simulink model "car_model"  (R2017a)
settings: Solver=VariableStepAuto  StartTime=0.0  StopTime=tf  RelTol=1e-3  AbsTol=1e-6
values from neighbouring files (symbols this model uses):
  MAX_DELTA_i = deg2rad(MAX_DELTA_i)    [run_sim.m]
  x0 = double(subs([qs0; ps0], symbs, vals))    [run_sim.m]
undefined symbols (not defined in the file or in its folder): sys
(part 2 of 2)

== matlab function car_model/Vehicle/Steering_model/Efforts/Constrained_efforts ==
  data: in1 input; in2 input; fs output
function fs = ConstrainedEffort(in1,in2)

%    This function was generated by the Symbolic Math Toolbox version 7.2.

%    28-Oct-2020 21:52:33



delta_i = in1(4,:);

delta_o = in1(5,:);

f_phi_i = in2(1,:);

f_phi_l = in2(4,:);

f_phi_o = in2(2,:);

f_phi_r = in2(3,:);

p1 = in1(10,:);

p2 = in1(11,:);

p3 = in1(12,:);

p4 = in1(13,:);

phi_i = in1(6,:);

phi_l = in1(9,:);

phi_o = in1(7,:);

phi_r = in1(8,:);

theta = in1(3,:);

t2 = p1.^2;

t3 = p4.^2;

t4 = theta.*2.0;

t5 = p3.^2;

t6 = delta_i.*2.0;

t7 = delta_o.*2.0;

t8 = phi_o.*2.0;

t9 = p2.^2;

t10 = t4+t7+t8;

t11 = sin(t10);

t12 = t4+t7-t8;

t13 = sin(t12);

t14 = phi_o.*4.0;

t15 = t4+t7+t14;

t16 = sin(t15);

t17 = sin(t4);

t18 = t4+t7;

t19 = sin(t18);

t20 = phi_l.*2.0;

t21 = phi_l.*4.0;

t22 = -t4+t20;

t23 = sin(t22);

t24 = t4+t20;

t25 = sin(t24);

t26 = phi_l.*3.0;

t27 = phi_r.*2.0;

t28 = phi_r.*4.0;

t29 = phi_i.*4.0;

t30 = delta_o-t14+theta;

t31 = sin(t30);

t32 = delta_o+t14+theta;

t33 = sin(t32);

t34 = phi_o.*3.0;

t35 = delta_o+theta;

t36 = sin(t35);

t37 = tan(delta_i);

t38 = t37.*(3.0./2.0);

t39 = t38+9.0./2.0;

t40 = 1.0./t39.^2;

t41 = t21+theta;

t42 = sin(t41);

t43 = t4+t7-t14;

t44 = sin(t43);

t45 = sin(t8);

t46 = sin(t14);

t47 = -t4+t27;

t48 = sin(t47);

t49 = t4+t27;

t50 = sin(t49);

t51 = phi_r.*3.0;

t52 = t21-theta;

t53 = sin(t52);

t54 = -t4+t21;

t55 = sin(t54);

t56 = t4+t21;

t57 = sin(t56);

t58 = cos(theta);

t59 = sin(theta);

t60 = phi_i.*2.0;

t64 = cos(t6);

t65 = t64.*(9.0./2.0);

t66 = sin(t6);

t67 = t66.*(3.0./2.0);

t61 = t65+t67+9.0./2.0;

t62 = t4+t6+t60;

t63 = sin(t62);

t68 = t61.^2;

t69 = cos(t7);

t70 = t69.*(9.0./2.0);

t71 = sin(t7);

t74 = t71.*(3.0./2.0);

t72 = t70-t74+9.0./2.0;

t73 = 1.0./t72.^2;

t75 = t4+t6+t29;

t76 = sin(t75);

t77 = t28+theta;

t78 = sin(t77);

t79 = t4+t6;

t80 = sin(t79);

t81 = delta_i-t29+theta;

t82 = sin(t81);

t83 = delta_i+t29+theta;

t84 = sin(t83);

t85 = 1.0./t39;

t86 = delta_i+theta;

t87 = sin(t86);

t88 = t28-theta;

t89 = sin(t88);

t90 = -t4+t28;

t91 = sin(t90);

t92 = t4+t28;

t93 = sin(t92);

t94 = 1.0./t72;

t95 = t4+t6-t60;

t96 = sin(t95);

t97 = t4+t6-t29;

t98 = sin(t97);

t99 = cos(delta_i);

t101 = t99.*9.0;

t102 = sin(delta_i);

t103 = t102.*(3.0./2.0);

t100 = t101-t103;

t104 = t99.^2;

t105 = cos(delta_o);

t106 = 1.0./t105.^2;

t107 = t100.^2;

t108 = t101+t103;

t109 = 1.0./t108.^2;

t110 = phi_i.*3.0;

t111 = 1.0./t105;

t112 = 1.0./t108;

t113 = sin(t60);

t114 = sin(t29);

t115 = phi_o+t4+t7;

t116 = sin(t115);

t117 = t5.*t116.*3.888459953911314e-2;

t118 = delta_o+phi_o+theta;

t119 = sin(t118);

t120 = -phi_o+t4+t7;

t121 = sin(t120);

t122 = t5.*t121.*3.888459953911314e-2;

t123 = t2.*t16.*6.480766589852189e-3;

t124 = t9.*t44.*6.480766589852189e-3;

t125 = t9.*t16.*6.480766589852189e-3;

t126 = t4+t7+t34;

t127 = sin(t126);

t128 = t2.*t19.*3.888459953911314e-2;

t129 = t9.*t19.*3.888459953911314e-2;

t130 = t5.*t19.*5.184613271881752e-2;

t131 = delta_o-phi_o+theta;

t132 = sin(t131);

t133 = t2.*t31.*1.296153317970438e-2;

t134 = t2.*t33.*1.296153317970438e-2;

t135 = t9.*t31.*1.296153317970438e-2;

t136 = t9.*t33.*1.296153317970438e-2;

t137 = delta_o-t34+theta;

t138 = sin(t137);

t139 = delta_o+t34+theta;

t140 = sin(t139);

t141 = p1.*p3.*t13.*5.184613271881752e-2;

t142 = p1.*p2.*t44.*1.296153317970438e-2;

t143 = p1.*p2.*t16.*1.296153317970438e-2;

t144 = p2.*p3.*t13.*5.184613271881752e-2;

t145 = p1.*p3.*t16.*2.592306635940876e-2;

t146 = p2.*p3.*t16.*2.592306635940876e-2;

t147 = p1.*p3.*t45.*1.03692265437635e-1;

t148 = p2.*p3.*t45.*1.03692265437635e-1;

t149 = p1.*p3.*t46.*1.555383981564525e-1;

t150 = p2.*p3.*t46.*1.555383981564525e-1;

t151 = t2.*t76.*6.480766589852189e-3;

t152 = t2.*t80.*3.888459953911314e-2;

t153 = t2.*t82.*1.296153317970438e-2;

t154 = t2.*t84.*1.296153317970438e-2;

t155 = t9.*t68.*t73.*t98.*6.480766589852189e-3;

t156 = t9.*t68.*t73.*t76.*6.480766589852189e-3;

t157 = t9.*t68.*t73.*t80.*3.888459953911314e-2;

t158 = t9.*t68.*t73.*t82.*1.296153317970438e-2;

t159 = t9.*t68.*t73.*t84.*1.296153317970438e-2;

t160 = p1.*p2.*t61.*t80.*t94.*7.776919907822627e-2;

t161 = p1.*p2.*t61.*t82.*t94.*2.592306635940876e-2;

t162 = p1.*p2.*t61.*t84.*t94.*2.592306635940876e-2;

t163 = p1.*p2.*t61.*t94.*t98.*1.296153317970438e-2;

t164 = p1.*p2.*t61.*t76.*t94.*1.296153317970438e-2;

t165 = t5.*t80.*t104.*t106.*t107.*t109.*5.184613271881752e-2;

t166 = delta_i-phi_i+theta;

t167 = sin(t166);

t168 = delta_i+t110+theta;

t169 = sin(t168);

t170 = phi_i+t4+t6;

t171 = sin(t170);

t172 = t5.*t104.*t106.*t107.*t109.*t171.*3.888459953911314e-2;

t173 = delta_i+phi_i+theta;

t174 = sin(t173);

t175 = -phi_i+t4+t6;

t176 = sin(t175);

t177 = t5.*t104.*t106.*t107.*t109.*t176.*3.888459953911314e-2;

t178 = t4+t6-t110;

t179 = sin(t178);

t180 = t4+t6+t110;

t181 = sin(t180);

t182 = p1.*p3.*t96.*t99.*t100.*t111.*t112.*5.184613271881752e-2;

t183 = p1.*p3.*t76.*t99.*t100.*t111.*t112.*2.592306635940876e-2;

t184 = p1.*p3.*t99.*t100.*t111.*t112.*t113.*1.03692265437635e-1;

t185 = p1.*p3.*t99.*t100.*t111.*t112.*t114.*1.555383981564525e-1;

t186 = p1.*p3.*t84.*t99.*t100.*t111.*t112.*1.03692265437635e-1;

t187 = p2.*p3.*t61.*t94.*t96.*t99.*t100.*t111.*t112.*5.184613271881752e-2;

t188 = p2.*p3.*t61.*t76.*t94.*t99.*t100.*t111.*t112.*2.592306635940876e-2;

t189 = p2.*p3.*t61.*t94.*t99.*t100.*t111.*t112.*t113.*1.03692265437635e-1;

t190 = p2.*p3.*t61.*t94.*t99.*t100.*t111.*t112.*t114.*1.555383981564525e-1;

t191 = p2.*p3.*t61.*t84.*t94.*t99.*t100.*t111.*t112.*1.03692265437635e-1;

t192 = p1.*p2.*t19.*7.776919907822627e-2;

t193 = p1.*p2.*t31.*2.592306635940876e-2;

t194 = p1.*p2.*t33.*2.592306635940876e-2;

t195 = p1.*p3.*t33.*1.03692265437635e-1;

t196 = p2.*p3.*t33.*1.03692265437635e-1;

t197 = sin(t34);

t198 = sin(delta_o);

t199 = cos(t4);

t200 = sin(phi_o);

t201 = sin(t110);

t202 = sin(phi_i);

t203 = cos(t60);

t204 = cos(t8);

t205 = t58.*(3.0./4.0);

t206 = t59.*(9.0./2.0);

t207 = t6+theta;

t208 = sin(t207);

t209 = t58.*(9.0./2.0);

t210 = t59.*(3.0./4.0);

t211 = cos(t207);

t212 = sin(phi_r);

t213 = t212.^2;

t214 = cos(phi_r);

t215 = t214.^2;

t216 = t58.^2;

t217 = t59.^2;

t218 = sin(phi_l);

t219 = t218.^2;

t220 = cos(phi_l);

t221 = t220.^2;

fs = [t117+t122+t123+t124+t125+t128+t129+t130+t133+t134+t135+t136+t141+t142+t143+t144+t145+t146+t147+t148+t149+t150+t151+t152+t153+t154+t155+t156+t157+t158+t159+t160+t161+t162+t163+t164+t165+t172+t177+t182+t183+t184+t185+t186+t187+t188+t189+t190+t191+t192+t193+t194+t195+t196-t2.*t11.*2.592306635940876e-2-t5.*t11.*2.592306635940876e-2-t5.*t13.*2.592306635940876e-2+t2.*t17.*7.776919907822627e-2+t3.*t17.*5.184613271881752e-2-t9.*t11.*2.592306635940876e-2-t9.*t13.*2.592306635940876e-2+t2.*t23.*2.592306635940876e-2+t3.*t23.*2.592306635940876e-2-t2.*t25.*2.592306635940876e-2-t3.*t25.*2.592306635940876e-2-t2.*t36.*2.592306635940876e-2+t2.*t42.*1.296153317970438e-2-t9.*t36.*2.592306635940876e-2+t2.*t48.*2.592306635940876e-2-t2.*t50.*2.592306635940876e-2-t2.*t53.*1.296153317970438e-2-t2.*t55.*6.480766589852189e-3+t2.*t57.*6.480766589852189e-3-t2.*t59.*5.184613271881752e-2-t2.*t63.*2.592306635940876e-2+t2.*t78.*1.296153317970438e-2-t2.*t87.*2.592306635940876e-2-t2.*t89.*1.296153317970438e-2-t2.*t91.*6.480766589852189e-3+t2.*t93.*6.480766589852189e-3-t5.*t119.*2.592306635940876e-2-t5.*t127.*3.888459953911314e-2-t5.*t132.*2.592306635940876e-2-t5.*t138.*7.776919907822627e-2-t5.*t140.*7.776919907822627e-2-t2.*sin(phi_i.*-2.0+t4+t6).*2.592306635940876e-2+t2.*sin(phi_i.*-4.0+t4+t6).*6.480766589852189e-3-t2.*sin(phi_o.*-2.0+t4+t7).*2.592306635940876e-2+t2.*sin(phi_o.*-4.0+t4+t7).*6.480766589852189e-3-t5.*sin(phi_o.*-3.0+t4+t7).*3.888459953911314e-2+t3.*sin(phi_l+t4).*3.888459953911314e-2-t3.*sin(phi_l+theta).*2.592306635940876e-2-t3.*sin(t4+t26).*3.888459953911314e-2-t3.*sin(t26+theta).*7.776919907822627e-2-t3.*sin(phi_l-t4).*3.888459953911314e-2+t3.*sin(phi_l-theta).*2.592306635940876e-2+t3.*sin(-t4+t26).*3.888459953911314e-2+t3.*sin(t26-theta).*7.776919907822627e-2-t3.*t40.*sin(t4+t51).*7.87413140667041e-1-t3.*t40.*sin(t51+theta).*1.574826281334082+p1.*p4.*sin(t20).*1.03692265437635e-1+p1.*p4.*sin(t21).*1.555383981564525e-1-t3.*t40.*sin(phi_r-t4).*7.87413140667041e-1+t3.*t40.*sin(phi_r-theta).*5.249420937780273e-1+t3.*t40.*sin(-t4+t51).*7.87413140667041e-1+t3.*t40.*sin(t51-theta).*1.574826281334082-t2.*t59.*(t209+t210).*4.24125e3-p1.*p2.*t11.*5.184613271881752e-2-p1.*p3.*t11.*5.184613271881752e-2-p1.*p2.*t13.*5.184613271881752e-2-p2.*p3.*t11.*5.184613271881752e-2-p1.*p4.*t23.*5.184613271881752e-2-p1.*p4.*t25.*5.184613271881752e-2-p1.*p3.*t31.*1.03692265437635e-1-p2.*p3.*t31.*1.03692265437635e-1-p1.*p2.*t36.*5.184613271881752e-2+p1.*p4.*t42.*1.03692265437635e-1-p1.*p3.*t44.*2.592306635940876e-2-p2.*p3.*t44.*2.592306635940876e-2+p1.*p4.*t53.*1.03692265437635e-1+p1.*p4.*t55.*2.592306635940876e-2+p1.*p4.*t57.*2.592306635940876e-2+t3.*t17.*t40.*1.049884187556055+t3.*t40.*t48.*5.249420937780273e-1-t3.*t40.*t50.*5.249420937780273e-1-t2.*t58.*(t205-t206).*4.24125e3+t3.*t40.*sin(phi_r+t4).*7.87413140667041e-1-t3.*t40.*sin(phi_r+theta).*5.249420937780273e-1-p1.*p4.*t48.*t85.*2.333075972346788e-1-p1.*p4.*t50.*t85.*2.333075972346788e-1+p1.*p4.*t78.*t85.*4.666151944693576e-1+p1.*p4.*t85.*t89.*4.666151944693576e-1+p1.*p4.*t85.*t91.*1.166537986173394e-1+p1.*p4.*t85.*t93.*1.166537986173394e-1-t9.*t63.*t68.*t73.*2.592306635940876e-2-t9.*t68.*t73.*t87.*2.592306635940876e-2-t9.*t68.*t73.*t96.*2.592306635940876e-2+p1.*p4.*t85.*sin(t27).*4.666151944693576e-1+p1.*p4.*t85.*sin(t28).*6.999227917040365e-1-p1.*p2.*t61.*t63.*t94.*5.184613271881752e-2-p1.*p2.*t61.*t87.*t94.*5.184613271881752e-2-p1.*p2.*t61.*t94.*t96.*5.184613271881752e-2-t5.*t63.*t104.*t106.*t107.*t109.*2.592306635940876e-2-t5.*t96.*t104.*t106.*t107.*t109.*2.592306635940876e-2-t5.*t104.*t106.*t107.*t109.*t167.*2.592306635940876e-2-t5.*t104.*t106.*t107.*t109.*t169.*7.776919907822627e-2-t5.*t104.*t106.*t107.*t109.*t174.*2.592306635940876e-2-t5.*t104.*t106.*t107.*t109.*t179.*3.888459953911314e-2-t5.*t104.*t106.*t107.*t109.*t181.*3.888459953911314e-2-t5.*t104.*t106.*t107.*t109.*sin(delta_i-phi_i.*3.0+theta).*7.776919907822627e-2-p1.*p3.*t63.*t99.*t100.*t111.*t112.*5.184613271881752e-2-p1.*p3.*t82.*t99.*t100.*t111.*t112.*1.03692265437635e-1-p1.*p3.*t98.*t99.*t100.*t111.*t112.*2.592306635940876e-2-p2.*p3.*t61.*t63.*t94.*t99.*t100.*t111.*t112.*5.184613271881752e-2-p2.*p3.*t61.*t82.*t94.*t99.*t100.*t111.*t112.*1.03692265437635e-1-p2.*p3.*t61.*t94.*t98.*t99.*t100.*t111.*t112.*2.592306635940876e-2;t117+t122+t123+t124+t125+t128+t129+t130+t133+t134+t135+t136+t141+t142+t143+t144+t145+t146+t147+t148+t149+t150+t192+t193+t194+t195+t196-t2.*t11.*2.592306635940876e-2-t2.*t13.*2.592306635940876e-2-t5.*t11.*2.592306635940876e-2-t5.*t13.*2.592306635940876e-2-t9.*t11.*2.592306635940876e-2-t9.*t13.*2.592306635940876e-2-t2.*t36.*2.592306635940876e-2-t9.*t36.*2.592306635940876e-2+t2.*t44.*6.480766589852189e-3-t5.*t119.*2.592306635940876e-2-t5.*t127.*3.888459953911314e-2-t5.*t132.*2.592306635940876e-2-t5.*t138.*7.776919907822627e-2-t5.*t140.*7.776919907822627e-2-t5.*sin(t4+t7-t34).*3.888459953911314e-2+t61.*t94.*(t151+t152+t153+t154+t155+t156+t157+t158+t159+t160+t161+t162+t163+t164+t165+t172+t177+t182+t183+t184+t185+t186+t187+t188+t189+t190+t191-t2.*t63.*2.592306635940876e-2-t2.*t87.*2.592306635940876e-2-t2.*t96.*2.592306635940876e-2+t2.*t98.*6.480766589852189e-3-t9.*t63.*t68.*t73.*2.592306635940876e-2-t9.*t68.*t73.*t87.*2.592306635940876e-2-t9.*t68.*t73.*t96.*2.592306635940876e-2-p1.*p2.*t61.*t63.*t94.*5.184613271881752e-2-p1.*p2.*t61.*t87.*t94.*5.184613271881752e-2-p1.*p2.*t61.*t94.*t96.*5.184613271881752e-2-t5.*t63.*t104.*t106.*t107.*t109.*2.592306635940876e-2-t5.*t96.*t104.*t106.*t107.*t109.*2.592306635940876e-2-t5.*t104.*t106.*t107.*t109.*t167.*2.592306635940876e-2-t5.*t104.*t106.*t107.*t109.*t169.*7.776919907822627e-2-t5.*t104.*t106.*t107.*t109.*t174.*2.592306635940876e-2-t5.*t104.*t106.*t107.*t109.*t179.*3.888459953911314e-2-t5.*t104.*t106.*t107.*t109.*t181.*3.888459953911314e-2-t5.*t104.*t106.*t107.*t109.*sin(delta_i-t110+theta).*7.776919907822627e-2-p1.*p3.*t63.*t99.*t100.*t111.*t112.*5.184613271881752e-2-p1.*p3.*t82.*t99.*t100.*t111.*t112.*1.03692265437635e-1-p1.*p3.*t98.*t99.*t100.*t111.*t112.*2.592306635940876e-2-p2.*p3.*t61.*t63.*t94.*t99.*t100.*t111.*t112.*5.184613271881752e-2-p2.*p3.*t61.*t82.*t94.*t99.*t100.*t111.*t112.*1.03692265437635e-1-p2.*p3.*t61.*t94.*t98.*t99.*t100.*t111.*t112.*2.592306635940876e-2)-p1.*p2.*t11.*5.184613271881752e-2-p1.*p3.*t11.*5.184613271881752e-2-p1.*p2.*t13.*5.184613271881752e-2-p2.*p3.*t11.*5.184613271881752e-2-p1.*p3.*t31.*1.03692265437635e-1-p2.*p3.*t31.*1.03692265437635e-1-p1.*p2.*t36.*5.184613271881752e-2-p1.*p3.*t44.*2.592306635940876e-2-p2.*p3.*t44.*2.592306635940876e-2;f_phi_o-t2.*t45.*5.184613271881752e-2-t2.*t46.*7.776919907822627e-2-t5.*t45.*5.184613271881752e-2-t9.*t45.*5.184613271881752e-2-t9.*t46.*7.776919907822627e-2-p1.*p2.*t45.*1.03692265437635e-1-p1.*p2.*t46.*1.555383981564525e-1-p1.*p3.*t17.*t69.*1.03692265437635e-1-p2.*p3.*t17.*t69.*1.03692265437635e-1-p1.*p3.*t71.*t199.*1.03692265437635e-1-p2.*p3.*t71.*t199.*1.03692265437635e-1-t2.*t17.*t45.*t71.*5.184613271881752e-2+t2.*t17.*t46.*t71.*2.592306635940876e-2-t5.*t17.*t45.*t71.*5.184613271881752e-2-t9.*t17.*t45.*t71.*5.184613271881752e-2+t9.*t17.*t46.*t71.*2.592306635940876e-2-t2.*t46.*t58.*t105.*1.03692265437635e-1-t9.*t46.*t58.*t105.*1.03692265437635e-1+t2.*t17.*t71.*t197.*5.184613271881752e-2-t2.*t17.*t71.*t200.*1.555383981564525e-1+t9.*t17.*t71.*t197.*5.184613271881752e-2-t9.*t17.*t71.*t200.*1.555383981564525e-1+t2.*t46.*t59.*t198.*1.03692265437635e-1+t9.*t46.*t59.*t198.*1.03692265437635e-1+t2.*t45.*t69.*t199.*5.184613271881752e-2-t2.*t46.*t69.*t199.*2.592306635940876e-2+t5.*t45.*t69.*t199.*5.184613271881752e-2+t9.*t45.*t69.*t199.*5.184613271881752e-2-t9.*t46.*t69.*t199.*2.592306635940876e-2-t2.*t58.*t105.*t197.*5.184613271881752e-2-t2.*t58.*t105.*t200.*5.184613271881752e-2-t9.*t58.*t105.*t197.*5.184613271881752e-2-t9.*t58.*t105.*t200.*5.184613271881752e-2+t2.*t59.*t197.*t198.*5.184613271881752e-2+t2.*t59.*t198.*t200.*5.184613271881752e-2+t9.*t59.*t197.*t198.*5.184613271881752e-2+t9.*t59.*t198.*t200.*5.184613271881752e-2-t2.*t69.*t197.*t199.*5.184613271881752e-2+t2.*t69.*t199.*t200.*1.555383981564525e-1-t9.*t69.*t197.*t199.*5.184613271881752e-2+t9.*t69.*t199.*t200.*1.555383981564525e-1-t99.*t100.*t111.*t112.*(t2.*t113.*5.184613271881752e-2+t2.*t114.*7.776919907822627e-2+t2.*t17.*t66.*t113.*5.184613271881752e-2-t2.*t17.*t66.*t114.*2.592306635940876e-2+t9.*t68.*t73.*t113.*5.184613271881752e-2+t9.*t68.*t73.*t114.*7.776919907822627e-2+t2.*t58.*t99.*t114.*1.03692265437635e-1-t2.*t59.*t102.*t114.*1.03692265437635e-1-t2.*t17.*t66.*t201.*5.184613271881752e-2+t2.*t17.*t66.*t202.*1.555383981564525e-1+t2.*t58.*t99.*t201.*5.184613271881752e-2+t2.*t58.*t99.*t202.*5.184613271881752e-2-t2.*t59.*t102.*t201.*5.184613271881752e-2-t2.*t59.*t102.*t202.*5.184613271881752e-2-t2.*t64.*t113.*t199.*5.184613271881752e-2+t2.*t64.*t114.*t199.*2.592306635940876e-2+t2.*t64.*t199.*t201.*5.184613271881752e-2-t2.*t64.*t199.*t202.*1.555383981564525e-1+p1.*p2.*t61.*t94.*t113.*1.03692265437635e-1+p1.*p2.*t61.*t94.*t114.*1.555383981564525e-1+t9.*t17.*t66.*t68.*t73.*t113.*5.184613271881752e-2-t9.*t17.*t66.*t68.*t73.*t114.*2.592306635940876e-2+t9.*t58.*t68.*t73.*t99.*t114.*1.03692265437635e-1-t9.*t59.*t68.*t73.*t102.*t114.*1.03692265437635e-1-t9.*t17.*t66.*t68.*t73.*t201.*5.184613271881752e-2+t9.*t17.*t66.*t68.*t73.*t202.*1.555383981564525e-1+t9.*t58.*t68.*t73.*t99.*t201.*5.184613271881752e-2+t9.*t58.*t68.*t73.*t99.*t202.*5.184613271881752e-2-t9.*t59.*t68.*t73.*t102.*t201.*5.184613271881752e-2-t9.*t59.*t68.*t73.*t102.*t202.*5.184613271881752e-2-t9.*t64.*t68.*t73.*t113.*t199.*5.184613271881752e-2+t9.*t64.*t68.*t73.*t114.*t199.*2.592306635940876e-2+t5.*t104.*t106.*t107.*t109.*t113.*5.184613271881752e-2+t9.*t64.*t68.*t73.*t199.*t201.*5.184613271881752e-2-t9.*t64.*t68.*t73.*t199.*t202.*1.555383981564525e-1+p1.*p2.*t17.*t61.*t66.*t94.*t113.*1.03692265437635e-1-p1.*p2.*t17.*t61.*t66.*t94.*t114.*5.184613271881752e-2+p1.*p2.*t58.*t61.*t94.*t99.*t114.*2.073845308752701e-1-p1.*p2.*t59.*t61.*t94.*t102.*t114.*2.073845308752701e-1-p1.*p2.*t17.*t61.*t66.*t94.*t201.*1.03692265437635e-1+p1.*p2.*t17.*t61.*t66.*t94.*t202.*3.110767963129051e-1+p1.*p2.*t58.*t61.*t94.*t99.*t201.*1.03692265437635e-1+p1.*p2.*t58.*t61.*t94.*t99.*t202.*1.03692265437635e-1-p1.*p2.*t59.*t61.*t94.*t102.*t201.*1.03692265437635e-1-p1.*p2.*t59.*t61.*t94.*t102.*t202.*1.03692265437635e-1-p1.*p2.*t61.*t64.*t94.*t113.*t199.*1.03692265437635e-1+p1.*p2.*t61.*t64.*t94.*t114.*t199.*5.184613271881752e-2+p1.*p2.*t61.*t64.*t94.*t199.*t201.*1.03692265437635e-1-p1.*p2.*t61.*t64.*t94.*t199.*t202.*3.110767963129051e-1+p1.*p3.*t17.*t64.*t99.*t100.*t111.*t112.*1.03692265437635e-1+p1.*p3.*t66.*t99.*t100.*t111.*t112.*t199.*1.03692265437635e-1+t5.*t17.*t66.*t104.*t106.*t107.*t109.*t113.*5.184613271881752e-2-t5.*t64.*t104.*t106.*t107.*t109.*t113.*t199.*5.184613271881752e-2-p1.*p3.*t17.*t64.*t99.*t100.*t111.*t112.*t203.*1.03692265437635e-1-p1.*p3.*t66.*t99.*t100.*t111.*t112.*t199.*t203.*1.03692265437635e-1+p2.*p3.*t17.*t61.*t64.*t94.*t99.*t100.*t111.*t112.*1.03692265437635e-1+p2.*p3.*t61.*t66.*t94.*t99.*t100.*t111.*t112.*t199.*1.03692265437635e-1-p2.*p3.*t17.*t61.*t64.*t94.*t99.*t100.*t111.*t112.*t203.*1.03692265437635e-1-p2.*p3.*t61.*t66.*t94.*t99.*t100.*t111.*t112.*t199.*t203.*1.03692265437635e-1)+f_phi_i.*t99.*t100.*t111.*t112-p1.*p2.*t17.*t45.*t71.*1.03692265437635e-1+p1.*p2.*t17.*t46.*t71.*5.184613271881752e-2-p1.*p2.*t46.*t58.*t105.*2.073845308752701e-1+p1.*p2.*t17.*t71.*t197.*1.03692265437635e-1-p1.*p2.*t17.*t71.*t200.*3.110767963129051e-1+p1.*p3.*t17.*t69.*t204.*1.03692265437635e-1+p2.*p3.*t17.*t69.*t204.*1.03692265437635e-1+p1.*p2.*t46.*t59.*t198.*2.073845308752701e-1+p1.*p2.*t45.*t69.*t199.*1.03692265437635e-1-p1.*p2.*t46.*t69.*t199.*5.184613271881752e-2-p1.*p2.*t58.*t105.*t197.*1.03692265437635e-1-p1.*p2.*t58.*t105.*t200.*1.03692265437635e-1+p1.*p2.*t59.*t197.*t198.*1.03692265437635e-1+p1.*p2.*t59.*t198.*t200.*1.03692265437635e-1-p1.*p2.*t69.*t197.*t199.*1.03692265437635e-1+p1.*p2.*t69.*t199.*t200.*3.110767963129051e-1+p1.*p3.*t71.*t199.*t204.*1.03692265437635e-1+p2.*p3.*t71.*t199.*t204.*1.03692265437635e-1-t2.*t59.*t99.*t111.*t112.*(t208.*(-3.0./4.0)+t209+t210+t211.*(9.0./2.0)).*1.46003419575e3+t2.*t58.*t99.*t111.*t112.*(-t205+t206+t208.*(9.0./2.0)+t211.*(3.0./4.0)).*1.46003419575e3;f_phi_l+f_phi_r.*t85.*(9.0./2.0)-t85.*(t2.*t212.*t216.*2.073845308752701e-1-t2.*t212.*t217.*2.073845308752701e-1+t2.*t58.*t212.*t215.*2.073845308752701e-1+t2.*t212.*t213.*t214.*2.073845308752701e-1-t2.*t212.*t213.*t216.*4.147690617505401e-1+t2.*t212.*t214.*t215.*6.221535926258102e-1+t2.*t212.*t213.*t217.*4.147690617505401e-1-t2.*t212.*t214.*t217.*2.073845308752701e-1-t2.*t212.*t215.*t216.*2.073845308752701e-1+t2.*t212.*t215.*t217.*2.073845308752701e-1-p1.*p4.*t58.*t59.*t85.*1.866460777877431+t3.*t40.*t212.*t214.*t217.*4.199536750224219-t2.*t58.*t212.*t213.*t214.*4.147690617505401e-1+t2.*t58.*t212.*t214.*t215.*4.147690617505401e-1-t2.*t212.*t213.*t214.*t216.*6.221535926258102e-1-t2.*t212.*t214.*t215.*t216.*2.073845308752701e-1+p1.*p4.*t58.*t59.*t85.*t213.*3.732921555754861+p1.*p4.*t58.*t59.*t85.*t215.*1.866460777877431).*(9.0./2.0)-t2.*t216.*t218.*2.073845308752701e-1+t2.*t217.*t218.*2.073845308752701e-1+p1.*p4.*t58.*t59.*4.147690617505401e-1-t2.*t58.*t218.*t221.*2.073845308752701e-1+t2.*t216.*t218.*t219.*4.147690617505401e-1-t2.*t217.*t218.*t219.*4.147690617505401e-1+t2.*t216.*t218.*t221.*2.073845308752701e-1+t2.*t217.*t218.*t220.*2.073845308752701e-1-t2.*t217.*t218.*t221.*2.073845308752701e-1-t3.*t217.*t218.*t220.*2.073845308752701e-1-t2.*t218.*t219.*t220.*2.073845308752701e-1-t2.*t218.*t220.*t221.*6.221535926258102e-1-p1.*p4.*t58.*t59.*t219.*8.295381235010802e-1-p1.*p4.*t58.*t59.*t221.*4.147690617505401e-1+t2.*t58.*t218.*t219.*t220.*4.147690617505401e-1-t2.*t58.*t218.*t220.*t221.*4.147690617505401e-1+t2.*t216.*t218.*t219.*t220.*6.221535926258102e-1+t2.*t216.*t218.*t220.*t221.*2.073845308752701e-1];

end

== matlab function car_model/Vehicle/Steering_model/Mass_block/H ==
  data: C_matrix input; H output; M input
function H = ConstrinedMassMatrix(C_matrix, M)
% MASSMATRIX
%    This function was generated by the Symbolic Math Toolbox version 7.2.
%    16-Oct-2020 11:55:07

    H = C_matrix'*M*C_matrix;
end

== matlab function car_model/Vehicle/Steering_model/Mass_block/invH ==
  data: matrix input; inv_matrix output
function inv_matrix = matrix_inverse(matrix)
% MASSMATRIX
%    This function was generated by the Symbolic Math Toolbox version 7.2.
%    16-Oct-2020 11:55:07

    inv_matrix = inv(matrix);
end

== matlab function car_model/Vehicle/Steering_model/Mass_block/inverse_matrix_ ==
  data: matrix input; inv_matrix output
function inv_matrix = matrix_inverse(matrix)
% MASSMATRIX
%    This function was generated by the Symbolic Math Toolbox version 7.2.
%    16-Oct-2020 11:55:07

    inv_matrix = inv(matrix);
end

== matlab function car_model/Vehicle/Steering_model/Mass_block/square_root_M ==
  data: matrix input; square_root_matrix output
function square_root_matrix = matrix_square_root(matrix)
% MASSMATRIX
%    This function was generated by the Symbolic Math Toolbox version 7.2.
%    16-Oct-2020 11:55:07

    square_root_matrix = real(sqrtm(matrix));
end

== matlab function car_model/Vehicle/Steering_model/Mass_block/inverse_matrix ==
  data: matrix input; inv_matrix output
function inv_matrix = matrix_inverse(matrix)
% MASSMATRIX
%    This function was generated by the Symbolic Math Toolbox version 7.2.
%    16-Oct-2020 11:55:07

    inv_matrix = inv(matrix);
end

== matlab function car_model/Vehicle/Steering_model/Auxiliary_matrices/C_p ==
  data: in1 input; qp output
function qp = KinematicVector(in1)

%    This function was generated by the Symbolic Math Toolbox version 7.2.

%    28-Oct-2020 21:52:11



delta_i = in1(4,:);

delta_o = in1(5,:);

p1 = in1(10,:);

p2 = in1(11,:);

p3 = in1(12,:);

p4 = in1(13,:);

theta = in1(3,:);

t2 = cos(delta_i);

t3 = cos(theta);

t4 = t3.*(9.0./2.0);

t5 = sin(theta);

t6 = t5.*(3.0./4.0);

t7 = delta_i.*2.0;

t8 = t7+theta;

t9 = cos(delta_o);

t10 = 1.0./t9;

t11 = t2.*9.0;

t12 = sin(delta_i);

t13 = t12.*(3.0./2.0);

t14 = t11+t13;

t15 = 1.0./t14;

t16 = sin(t8);

t17 = t3.*(3.0./4.0);

t18 = t5.*(9.0./2.0);

t19 = cos(t8);

t20 = delta_o.*2.0;

qp = [p1.*(t4+t6)+p3.*t2.*t10.*t15.*(t4+t6-t16.*(3.0./4.0)+t19.*(9.0./2.0)).*3.442462000000001e-1;-p1.*(t17-t18)+p3.*t2.*t10.*t15.*(t16.*(9.0./2.0)-t17+t18+t19.*(3.0./4.0)).*3.442462000000001e-1;p1;(p2.*(cos(t7).*(9.0./2.0)+sin(t7).*(3.0./2.0)+9.0./2.0))./(cos(t20).*(9.0./2.0)-sin(t20).*(3.0./2.0)+9.0./2.0);p2;p3.*t2.*t10.*t15.*(t11-t13);p3;(p4.*(9.0./2.0))./(tan(delta_i).*(3.0./2.0)+9.0./2.0);p4];

end
